simulink model "ROSCO_v1"  (R2023a)
settings: Solver=ode4  StartTime=0.0  StopTime=TMax  FixedStep=simu.dt  RelTol=1e-3  EnableMultiTasking=on
undefined symbols (not defined in the file): Azimuth_list, DiscIntNeverNeededParam, F, n_FixFrameInputs, n_FixFrameOutputs, n_RotTripletInputs, n_RotTripletOutputs, new_seq_inp, new_seq_out, OutList, Parameter, R, rpm2radps, simu, StateSpace, strmatch
libraries: simulink x10
(part 2 of 3)

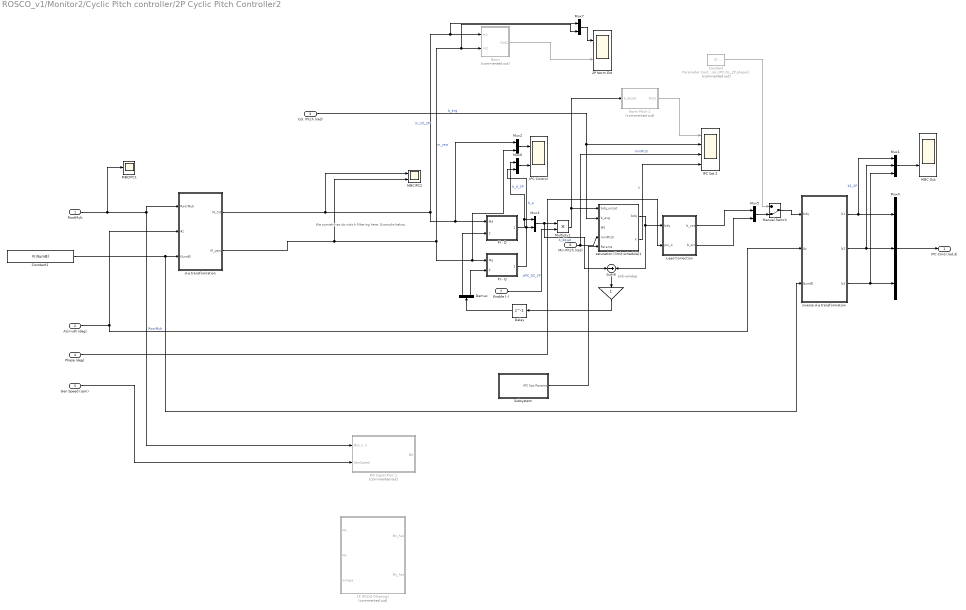
== system ROSCO_v1/Monitor2/Cyclic Pitch controller/2P Cyclic Pitch Controller2 ==
  note: We sometimes do notch filtering here. Example below.
  note: anti-windup
  note: k
  RootMyb : Inport
  Azimuth (deg) : Inport  Port=2
  Col. Pitch (rad) : Inport  Port=3
  Phase (deg) : Inport  Port=4
  Gen Speed (rpm) : Inport  Port=5
  Min Pitch (rad) : Inport  Port=6
  Enable (-) : Inport  Port=7
  " " : Gain
  1P IPCDQ Filtering1 : Subsystem  Commented=on
  2P Norm Est : Scope  NumInputPorts=2
  Constant : Constant  Commented=on  Value=Parameter.Control.cIPC.OL_2P.amp * [cosd(Parameter.Control.cIPC.OL_2P.phase), sind(Parameter.Control.cIPC.OL_2P.phase)]
  Constant1 : Constant  Value=R.NumBl
  Delay : Delay  DelayLength=1
  Demux : Demux  Outputs=2
  IPC Control : Scope  NumInputPorts=2
  IPC Sat 2 : Scope  NumInputPorts=4
  Lead Correction : MATLAB Function  TreatAsAtomicUnit=on
  M0 Signal Proc.1 : Subsystem  Commented=on
  MBC Out : Scope  NumInputPorts=2
  MBCIPC1 : Scope
  MBCIPC2 : Scope  NumInputPorts=2
  Manual Switch : ManualSwitch  CurrentSetting=0
  Multiply1 : Product
  Mux1 : Mux  Inputs=3
  Mux{2..3,5..7} (5 alike) : Mux  Inputs=2
  Mux4 : Mux  Inputs=3
  Norm : Subsystem  Commented=on
  Norm Pitch 2 : Subsystem  Commented=on
  PI - D : Subsystem  TreatAsAtomicUnit=on  SystemSampleTime=simu.dt
      settings: MinAlgLoopOccurrences=on
  PI - Q : Subsystem  TreatAsAtomicUnit=on  SystemSampleTime=simu.dt
      settings: MinAlgLoopOccurrences=on
  Subsystem : Subsystem
  Sum9 : Sum  Inputs=-|+
  d-q transformation : MATLAB Function  TreatAsAtomicUnit=on
  inverse d-q transformation : MATLAB Function  TreatAsAtomicUnit=on
  saturation (limit schedule)1 : MATLAB Function  TreatAsAtomicUnit=on
  IPC Cmd (rad,3) : Outport  VectorParamsAs1DForOutWhenUnconnected=off
  wires:
  Enable (-)/1 -> Multiply1/2  "cIPC_GS_2P"
  Norm Pitch 2/1(Out1) -> IPC Sat 2/1
  Min Pitch (rad)/1 -> saturation (limit schedule)1/4(minPitch), IPC Sat 2/3  "minPitch"
  Norm/1(Out1) -> 2P Norm Est/2
  Mux7/1 -> 2P Norm Est/1
  Mux2/1 -> IPC Control/1
  Mux6/1 -> IPC Control/2
  Mux1/1 -> MBC Out/2
  d-q transformation/2(M_yaw) -> PI - Q/1(Mq), Mux2/2, Norm/2(In2), Mux7/2, MBCIPC2/2  "m_yaw"
  Constant1/1 -> inverse d-q transformation/3(NumBl), d-q transformation/3(NumBl)
  saturation (limit schedule)1/2(k) -> IPC Sat 2/4
  Lead Correction/2(b_sin) -> Mux5/2
  Lead Correction/1(b_cos) -> Mux5/1
  Azimuth (deg)/1 -> inverse d-q transformation/2(Az), d-q transformation/2(Az)
  Sum9/1 -> " "/1
  RootMyb/1 -> MBCIPC1/1, M0 Signal Proc.1/1("My1,2, 3"), d-q transformation/1(RootMyb)  "RootMyb"
  " "/1 -> Delay/1
  Delay/1 -> Demux/1
  Mux4/1 -> IPC Cmd (rad,3)/1
  inverse d-q transformation/2(b2) -> Mux4/2, Mux1/2
  Demux/2 -> PI - Q/2(Anti-windup)
  inverse d-q transformation/1(b1) -> Mux4/1, Mux1/1  "b1_2P"
  Demux/1 -> PI - D/2(Anti-windup)
  PI - D/1(Theta_tilt) -> Mux6/1, Mux3/1  "b_d_2P"
  PI - Q/1(Theta_yaw) -> Mux6/2, Mux3/2  "b_q"
  Phase (deg)/1 -> Lead Correction/2(psi_o)
  inverse d-q transformation/3(b3) -> Mux4/3, Mux1/3
  d-q transformation/1(M_tilt) -> PI - D/1(Md), Mux2/1, Norm/1(In1), Mux7/1, MBCIPC2/1  "m_tilt_2P"
  Gen Speed (rpm)/1 -> M0 Signal Proc.1/2(GenSpeed)
  saturation (limit schedule)1/1(bdq) -> Lead Correction/1(bdq), Sum9/2
  Col. Pitch (rad)/1 -> IPC Sat 2/2, saturation (limit schedule)1/2(b_avg)  "b_avg"
  Subsystem/1(IPC Sat Params) -> saturation (limit schedule)1/5(Params)
  Mux3/1 -> Sum9/1, Multiply1/1  "b_dqsat"
  Multiply1/1 -> Norm Pitch 2/1(b_dqsat), saturation (limit schedule)1/1(bdq_unsat)
  Mux5/1 -> Manual Switch/2
  Manual Switch/1 -> inverse d-q transformation/1(bdq)
  Constant/1 -> Manual Switch/1

== system ROSCO_v1/Torque Controller/VS_OmegaRef/Omega_opt ==
  note: % Assuming known wind speed, initially, and not using GenSpeed
  TSR_opt : Inport
  Wind Speed : Inport  Port=2
  Divide : Product  Inputs=*/
  Multiply : Product
  "Rot -> GenSpeed" : Gain  Gain=R.GBRatio
  Rotor Radius : Constant  Value=R.RotorRad
  Omega_opt : Outport  VectorParamsAs1DForOutWhenUnconnected=off
  wires:
  TSR_opt/1 -> Multiply/1
  Wind Speed/1 -> Multiply/2
  Multiply/1 -> Divide/1
  Rotor Radius/1 -> Divide/2
  Divide/1 -> "Rot -> GenSpeed"/1
  "Rot -> GenSpeed"/1 -> Omega_opt/1

== system ROSCO_v1/Monitor2/Cyclic Pitch controller/1P Cyclic Pitch Controller1/1P IPCDQ Filtering1 ==
  Mx : Inport
  My : Inport  Port=2
  omega : Inport  Port=3
  Discrete Filter2 : DiscreteFilter  Numerator=Parameter.Control.cIPC.IPCDQ_LPF.Numerator{1}  Denominator=Parameter.Control.cIPC.IPCDQ_LPF.Denominator{1}  SampleTime=Parameter.Control.DT
  Discrete Filter3 : DiscreteFilter  Numerator=Parameter.Control.cIPC.IPCDQ_LPF.Numerator{1}  Denominator=Parameter.Control.cIPC.IPCDQ_LPF.Denominator{1}  SampleTime=Parameter.Control.DT
  IPC NFs Man 2 : Scope  NumInputPorts=2
  Moving 3P Notch Man Y : Subsystem
  Moving 3P Notch Man Z : Subsystem
  Moving 6P Notch Man Y : Subsystem
  Moving 6P Notch Man Z : Subsystem
  Mux : Mux  Inputs=2
  Mux1 : Mux  Inputs=2
  Mx_hat : Outport  VectorParamsAs1DForOutWhenUnconnected=off
  My_hat : Outport  Port=2  VectorParamsAs1DForOutWhenUnconnected=off
  wires:
  omega/1 -> Moving 6P Notch Man Y/2(GenSpeedIN), Moving 3P Notch Man Y/2(GenSpeedIN), Moving 6P Notch Man Z/2(GenSpeedIN), Moving 3P Notch Man Z/2(GenSpeedIN)
  Mx/1 -> Mux/1, Moving 3P Notch Man Y/1(Input)
  My/1 -> Mux1/1, Moving 3P Notch Man Z/1(Input)
  Moving 6P Notch Man Z/1(Output) -> Discrete Filter3/1
  Moving 6P Notch Man Y/1(Output) -> Discrete Filter2/1
  Moving 3P Notch Man Y/1(Output) -> Moving 6P Notch Man Y/1(Input)
  Moving 3P Notch Man Z/1(Output) -> Moving 6P Notch Man Z/1(Input)
  Mux1/1 -> IPC NFs Man 2/2
  Mux/1 -> IPC NFs Man 2/1
  Discrete Filter3/1 -> Mux1/2, My_hat/1
  Discrete Filter2/1 -> Mux/2, Mx_hat/1

== system ROSCO_v1/Monitor2/Cyclic Pitch controller/1P Cyclic Pitch Controller1/M0 Signal Proc.1 ==
  "My1,2, 3" : Inport
  GenSpeed : Inport  Port=2
  Add : Sum  Inputs=+++
  Demux1 : Demux  Outputs=3
  Discrete Filter : DiscreteFilter  Numerator=Parameter.Control.cIPC.PSM0_LPF.Numerator{1}  Denominator=Parameter.Control.cIPC.PSM0_LPF.Denominator{1}  a0EqualsOne=on
  Gain : Gain  Gain=1/3
  Moving 1P Notch Man : Subsystem
  Moving 3P Notch Man : Subsystem
  Mux : Mux  Inputs=2
  Scope : Scope  NumInputPorts=2
  M0 : Outport  VectorParamsAs1DForOutWhenUnconnected=off
  wires:
  Demux1/1 -> Add/1
  Demux1/2 -> Add/2
  Add/1 -> Gain/1
  "My1,2, 3"/1 -> Demux1/1
  GenSpeed/1 -> Moving 3P Notch Man/2(GenSpeedIN), Moving 1P Notch Man/2(GenSpeedIN)
  Demux1/3 -> Add/3
  Moving 1P Notch Man/1(Output) -> Moving 3P Notch Man/1(Input)
  Mux/1 -> Scope/2
  Gain/1 -> Scope/1, Moving 1P Notch Man/1(Input)
  Moving 3P Notch Man/1(Output) -> Discrete Filter/1
  Discrete Filter/1 -> Mux/1, M0/1

== system ROSCO_v1/Monitor2/Cyclic Pitch controller/1P Cyclic Pitch Controller1/Norm ==
  In1 : Inport
  In2 : Inport  Port=2
  Add : Sum
  Discrete Filter1 : DiscreteFilter  Numerator=Parameter.Control.cIPC.IPCDQ_LPF.num{1}  Denominator=Parameter.Control.cIPC.IPCDQ_LPF.den{1}  SampleTime=Parameter.Control.DT
  Product : Product
  Product1 : Product
  Sqrt : Sqrt
  Out1 : Outport  VectorParamsAs1DForOutWhenUnconnected=off
  wires:
  Product/1 -> Add/1
  Product1/1 -> Add/2
  Sqrt/1 -> Discrete Filter1/1
  Add/1 -> Sqrt/1
  In2/1 -> Product1/1, Product1/2
  In1/1 -> Product/1, Product/2
  Discrete Filter1/1 -> Out1/1

== system ROSCO_v1/Monitor2/Cyclic Pitch controller/1P Cyclic Pitch Controller1/Norm Pitch ==
  b_dqsat : Inport
  Demux1 : Demux  Outputs=2
  Sqrt : Sqrt
  Square : Math  Operator=square  SignedPower=on
  Square1 : Math  Operator=square  SignedPower=on
  Sum : Sum
  Out1 : Outport  VectorParamsAs1DForOutWhenUnconnected=off
  wires:
  Demux1/1 -> Square/1
  Square1/1 -> Sum/2
  b_dqsat/1 -> Demux1/1
  Sum/1 -> Sqrt/1
  Demux1/2 -> Square1/1
  Square/1 -> Sum/1
  Sqrt/1 -> Out1/1

== system ROSCO_v1/Monitor2/Cyclic Pitch controller/1P Cyclic Pitch Controller1/PI - D ==
  Md : Inport
  Anti-windup : Inport  Port=2
  Discrete Derivative : simulink/Discrete/Discrete Derivative  gainval=1.0  ICPrevScaledInput=0.0  OutMin=[]  OutMax=[]  OutDataType=fixdt(1, 16)  OutScaling=2^-10  DoSatur=off
  Discrete Filter1 : DiscreteFilter  Commented=through  Numerator=Parameter.Control.cIPC.IPCDQ_LPF.num{1}  Denominator=Parameter.Control.cIPC.IPCDQ_LPF.den{1}  SampleTime=Parameter.Control.DT
  Integrator : DiscreteIntegrator  IntegratorMethod=Integration: Backward Euler  gainval=1  SampleTime=simu.dt  UpperSaturationLimit=1.570796/(.008068634/9.5492966)/(1./(1.+pi/2/.109997))  LowerSaturationLimit=0  ICPrevOutput=DiscIntNeverNeededParam  ICPrevScaledInput=DiscIntNeverNeededParam
  Kd : Gain  Gain=0
  Ki : Gain  Gain=R.IPC_KI_2P
  Kp : Gain  Gain=R.IPC_KP_1P
  Scope : Scope  NumInputPorts=2
  Sum3 : Sum  Inputs=+++
  Sum8 : Sum  Inputs=|++
  Theta_tilt : Outport  VectorParamsAs1DForOutWhenUnconnected=off
  wires:
  Ki/1 -> Sum8/1
  Sum3/1 -> Scope/1, Theta_tilt/1
  Md/1 -> Ki/1, Kp/1, Discrete Filter1/1
  Anti-windup/1 -> Scope/2, Sum8/2
  Sum8/1 -> Integrator/1
  Kd/1 -> Discrete Derivative/1
  Kp/1 -> Sum3/2
  Discrete Derivative/1 -> Sum3/1
  Integrator/1 -> Sum3/3
  Discrete Filter1/1 -> Kd/1

== system ROSCO_v1/Monitor2/Cyclic Pitch controller/1P Cyclic Pitch Controller1/PI - Q ==
  Mq : Inport
  Anti-windup : Inport  Port=2
  Discrete Derivative : simulink/Discrete/Discrete Derivative  gainval=1.0  ICPrevScaledInput=0.0  OutMin=[]  OutMax=[]  OutDataType=fixdt(1, 16)  OutScaling=2^-10  DoSatur=off
  Discrete Filter1 : DiscreteFilter  Commented=through  Numerator=Parameter.Control.cIPC.IPCDQ_LPF.num{1}  Denominator=Parameter.Control.cIPC.IPCDQ_LPF.den{1}  SampleTime=Parameter.Control.DT
  Integrator1 : DiscreteIntegrator  IntegratorMethod=Integration: Backward Euler  gainval=1  SampleTime=simu.dt  UpperSaturationLimit=1.570796/(.008068634/9.5492966)/(1./(1.+pi/2/.109997))  LowerSaturationLimit=0  ICPrevOutput=DiscIntNeverNeededParam  ICPrevScaledInput=DiscIntNeverNeededParam
  Kd : Gain  Gain=0
  Ki : Gain  Gain=R.IPC_KI_1P
  Kp : Gain  Gain=R.IPC_KP_1P
  Sum10 : Sum  Inputs=|++
  Sum3 : Sum  Inputs=+++
  Theta_yaw : Outport  VectorParamsAs1DForOutWhenUnconnected=off
  wires:
  Sum3/1 -> Theta_yaw/1
  Sum10/1 -> Integrator1/1
  Anti-windup/1 -> Sum10/2
  Integrator1/1 -> Sum3/3
  Ki/1 -> Sum10/1
  Kp/1 -> Sum3/2
  Mq/1 -> Discrete Filter1/1, Kp/1, Ki/1
  Kd/1 -> Discrete Derivative/1
  Discrete Derivative/1 -> Sum3/1
  Discrete Filter1/1 -> Kd/1

== system ROSCO_v1/Monitor2/Cyclic Pitch controller/1P Cyclic Pitch Controller1/Subsystem1 ==
  Constant3 : Constant
  Constant4 : Constant  Value=0
  Constant5 : Constant  Value=0
  Mux : Mux  Inputs=3
  IPC Sat Params : Outport  VectorParamsAs1DForOutWhenUnconnected=off
  wires:
  Constant3/1 -> Mux/1
  Constant4/1 -> Mux/2
  Constant5/1 -> Mux/3
  Mux/1 -> IPC Sat Params/1

== system ROSCO_v1/Monitor2/Cyclic Pitch controller/2P Cyclic Pitch Controller2/1P IPCDQ Filtering1 ==
  Mx : Inport
  My : Inport  Port=2
  omega : Inport  Port=3
  Discrete Filter2 : DiscreteFilter  Numerator=Parameter.Control.cIPC.IPCDQ_LPF.Numerator{1}  Denominator=Parameter.Control.cIPC.IPCDQ_LPF.Denominator{1}  SampleTime=Parameter.Control.DT
  Discrete Filter3 : DiscreteFilter  Numerator=Parameter.Control.cIPC.IPCDQ_LPF.Numerator{1}  Denominator=Parameter.Control.cIPC.IPCDQ_LPF.Denominator{1}  SampleTime=Parameter.Control.DT
  IPC NFs Man 2 : Scope  NumInputPorts=2
  Moving 3P Notch Man Y : Subsystem
  Moving 3P Notch Man Z : Subsystem
  Moving 6P Notch Man Y : Subsystem
  Moving 6P Notch Man Z : Subsystem
  Mux : Mux  Inputs=2
  Mux1 : Mux  Inputs=2
  Mx_hat : Outport  VectorParamsAs1DForOutWhenUnconnected=off
  My_hat : Outport  Port=2  VectorParamsAs1DForOutWhenUnconnected=off
  wires:
  omega/1 -> Moving 6P Notch Man Y/2(GenSpeedIN), Moving 3P Notch Man Y/2(GenSpeedIN), Moving 6P Notch Man Z/2(GenSpeedIN), Moving 3P Notch Man Z/2(GenSpeedIN)
  Mx/1 -> Mux/1, Moving 3P Notch Man Y/1(Input)
  My/1 -> Mux1/1, Moving 3P Notch Man Z/1(Input)
  Moving 6P Notch Man Z/1(Output) -> Discrete Filter3/1
  Moving 6P Notch Man Y/1(Output) -> Discrete Filter2/1
  Moving 3P Notch Man Y/1(Output) -> Moving 6P Notch Man Y/1(Input)
  Moving 3P Notch Man Z/1(Output) -> Moving 6P Notch Man Z/1(Input)
  Mux1/1 -> IPC NFs Man 2/2
  Mux/1 -> IPC NFs Man 2/1
  Discrete Filter3/1 -> Mux1/2, My_hat/1
  Discrete Filter2/1 -> Mux/2, Mx_hat/1

== system ROSCO_v1/Monitor2/Cyclic Pitch controller/2P Cyclic Pitch Controller2/M0 Signal Proc.1 ==
  "My1,2, 3" : Inport
  GenSpeed : Inport  Port=2
  Add : Sum  Inputs=+++
  Demux1 : Demux  Outputs=3
  Discrete Filter : DiscreteFilter  Numerator=Parameter.Control.cIPC.PSM0_LPF.Numerator{1}  Denominator=Parameter.Control.cIPC.PSM0_LPF.Denominator{1}  a0EqualsOne=on
  Gain : Gain  Gain=1/3
  Moving 1P Notch Man : Subsystem
  Moving 3P Notch Man : Subsystem
  Mux : Mux  Inputs=2
  Scope : Scope  NumInputPorts=2
  M0 : Outport  VectorParamsAs1DForOutWhenUnconnected=off
  wires:
  Demux1/1 -> Add/1
  Demux1/2 -> Add/2
  Add/1 -> Gain/1
  "My1,2, 3"/1 -> Demux1/1
  GenSpeed/1 -> Moving 3P Notch Man/2(GenSpeedIN), Moving 1P Notch Man/2(GenSpeedIN)
  Demux1/3 -> Add/3
  Moving 1P Notch Man/1(Output) -> Moving 3P Notch Man/1(Input)
  Mux/1 -> Scope/2
  Gain/1 -> Scope/1, Moving 1P Notch Man/1(Input)
  Moving 3P Notch Man/1(Output) -> Discrete Filter/1
  Discrete Filter/1 -> Mux/1, M0/1

== system ROSCO_v1/Monitor2/Cyclic Pitch controller/2P Cyclic Pitch Controller2/Norm ==
  In1 : Inport
  In2 : Inport  Port=2
  Add : Sum
  Discrete Filter1 : DiscreteFilter  Numerator=Parameter.Control.cIPC.IPCDQ_LPF.num{1}  Denominator=Parameter.Control.cIPC.IPCDQ_LPF.den{1}  SampleTime=Parameter.Control.DT
  Product : Product
  Product1 : Product
  Sqrt : Sqrt
  Out1 : Outport  VectorParamsAs1DForOutWhenUnconnected=off
  wires:
  Discrete Filter1/1 -> Out1/1
  In1/1 -> Product/2, Product/1
  In2/1 -> Product1/2, Product1/1
  Add/1 -> Sqrt/1
  Sqrt/1 -> Discrete Filter1/1
  Product1/1 -> Add/2
  Product/1 -> Add/1

== system ROSCO_v1/Monitor2/Cyclic Pitch controller/2P Cyclic Pitch Controller2/Norm Pitch 2 ==
  b_dqsat : Inport
  Demux1 : Demux  Outputs=2
  Sqrt : Sqrt
  Square : Math  Operator=square  SignedPower=on
  Square1 : Math  Operator=square  SignedPower=on
  Sum : Sum
  Out1 : Outport  VectorParamsAs1DForOutWhenUnconnected=off
  wires:
  Sqrt/1 -> Out1/1
  Square/1 -> Sum/1
  Demux1/2 -> Square1/1
  Sum/1 -> Sqrt/1
  b_dqsat/1 -> Demux1/1
  Square1/1 -> Sum/2
  Demux1/1 -> Square/1

== system ROSCO_v1/Monitor2/Cyclic Pitch controller/2P Cyclic Pitch Controller2/PI - D ==
  Md : Inport
  Anti-windup : Inport  Port=2
  Discrete Derivative : simulink/Discrete/Discrete Derivative  gainval=1.0  ICPrevScaledInput=0.0  OutMin=[]  OutMax=[]  OutDataType=fixdt(1, 16)  OutScaling=2^-10  DoSatur=off
  Discrete Filter1 : DiscreteFilter  Commented=through  Numerator=Parameter.Control.cIPC.IPCDQ_LPF.num{1}  Denominator=Parameter.Control.cIPC.IPCDQ_LPF.den{1}  SampleTime=Parameter.Control.DT
  Integrator : DiscreteIntegrator  IntegratorMethod=Integration: Backward Euler  gainval=1  SampleTime=simu.dt  UpperSaturationLimit=1.570796/(.008068634/9.5492966)/(1./(1.+pi/2/.109997))  LowerSaturationLimit=0  ICPrevOutput=DiscIntNeverNeededParam  ICPrevScaledInput=DiscIntNeverNeededParam
  Kd : Gain  Gain=0
  Ki : Gain  Gain=R.IPC_KI_2P
  Kp : Gain  Gain=R.IPC_KP_2P
  Sum3 : Sum  Inputs=+++
  Sum8 : Sum  Inputs=|++
  Theta_tilt : Outport  VectorParamsAs1DForOutWhenUnconnected=off
  wires:
  Discrete Filter1/1 -> Kd/1
  Integrator/1 -> Sum3/3
  Discrete Derivative/1 -> Sum3/1
  Kp/1 -> Sum3/2
  Kd/1 -> Discrete Derivative/1
  Sum8/1 -> Integrator/1
  Anti-windup/1 -> Sum8/2
  Md/1 -> Discrete Filter1/1, Kp/1, Ki/1
  Sum3/1 -> Theta_tilt/1
  Ki/1 -> Sum8/1

== system ROSCO_v1/Monitor2/Cyclic Pitch controller/2P Cyclic Pitch Controller2/PI - Q ==
  Mq : Inport
  Anti-windup : Inport  Port=2
  Discrete Derivative : simulink/Discrete/Discrete Derivative  gainval=1.0  ICPrevScaledInput=0.0  OutMin=[]  OutMax=[]  OutDataType=fixdt(1, 16)  OutScaling=2^-10  DoSatur=off
  Discrete Filter1 : DiscreteFilter  Commented=through  Numerator=Parameter.Control.cIPC.IPCDQ_LPF.num{1}  Denominator=Parameter.Control.cIPC.IPCDQ_LPF.den{1}  SampleTime=Parameter.Control.DT
  Integrator1 : DiscreteIntegrator  IntegratorMethod=Integration: Backward Euler  gainval=1  SampleTime=simu.dt  UpperSaturationLimit=1.570796/(.008068634/9.5492966)/(1./(1.+pi/2/.109997))  LowerSaturationLimit=0  ICPrevOutput=DiscIntNeverNeededParam  ICPrevScaledInput=DiscIntNeverNeededParam
  Kd : Gain  Gain=0
  Ki : Gain  Gain=R.IPC_KI_2P
  Kp : Gain  Gain=R.IPC_KP_2P
  Sum10 : Sum  Inputs=|++
  Sum3 : Sum  Inputs=+++
  Theta_yaw : Outport  VectorParamsAs1DForOutWhenUnconnected=off
  wires:
  Discrete Filter1/1 -> Kd/1
  Discrete Derivative/1 -> Sum3/1
  Kd/1 -> Discrete Derivative/1
  Mq/1 -> Ki/1, Kp/1, Discrete Filter1/1
  Kp/1 -> Sum3/2
  Ki/1 -> Sum10/1
  Integrator1/1 -> Sum3/3
  Anti-windup/1 -> Sum10/2
  Sum10/1 -> Integrator1/1
  Sum3/1 -> Theta_yaw/1

== system ROSCO_v1/Monitor2/Cyclic Pitch controller/2P Cyclic Pitch Controller2/Subsystem ==
  Constant3 : Constant
  Constant4 : Constant  Value=0
  Constant5 : Constant  Value=0
  Mux : Mux  Inputs=3
  IPC Sat Params : Outport  VectorParamsAs1DForOutWhenUnconnected=off
  wires:
  Constant3/1 -> Mux/1
  Constant4/1 -> Mux/2
  Constant5/1 -> Mux/3
  Mux/1 -> IPC Sat Params/1

== system ROSCO_v1/Monitor2/Cyclic Pitch controller/1P Cyclic Pitch Controller1/1P IPCDQ Filtering1/Moving 3P Notch Man Y ==
  Input : Inport
  GenSpeedIN : Inport  Port=2
  Gain : Gain  Gain=1/Parameter.Turbine.G * rpm2radps(1) * 3
  Moving 3P Filt Manual : Subsystem
  Slow Low Pass for Param : DiscreteStateSpace  A=Parameter.Control.cIPC.dLPF_slow.a  B=Parameter.Control.cIPC.dLPF_slow.b  C=Parameter.Control.cIPC.dLPF_slow.c  D=Parameter.Control.cIPC.dLPF_slow.d  SampleTime=Parameter.Control.DT
  Output : Outport  VectorParamsAs1DForOutWhenUnconnected=off
  wires:
  Slow Low Pass for Param/1 -> Gain/1
  Gain/1 -> Moving 3P Filt Manual/2(rot speed (rad/s))
  Input/1 -> Moving 3P Filt Manual/1(u)
  GenSpeedIN/1 -> Slow Low Pass for Param/1
  Moving 3P Filt Manual/1(Out1) -> Output/1

== system ROSCO_v1/Monitor2/Cyclic Pitch controller/1P Cyclic Pitch Controller1/1P IPCDQ Filtering1/Moving 3P Notch Man Z ==
  Input : Inport
  GenSpeedIN : Inport  Port=2
  Gain : Gain  Gain=1/Parameter.Turbine.G * rpm2radps(1) * 3
  Moving 3P Filt Manual : Subsystem
  Slow Low Pass for Param : DiscreteStateSpace  A=Parameter.Control.cIPC.dLPF_slow.a  B=Parameter.Control.cIPC.dLPF_slow.b  C=Parameter.Control.cIPC.dLPF_slow.c  D=Parameter.Control.cIPC.dLPF_slow.d  SampleTime=Parameter.Control.DT
  Output : Outport  VectorParamsAs1DForOutWhenUnconnected=off
  wires:
  Moving 3P Filt Manual/1(Out1) -> Output/1
  GenSpeedIN/1 -> Slow Low Pass for Param/1
  Input/1 -> Moving 3P Filt Manual/1(u)
  Gain/1 -> Moving 3P Filt Manual/2(rot speed (rad/s))
  Slow Low Pass for Param/1 -> Gain/1

== system ROSCO_v1/Monitor2/Cyclic Pitch controller/1P Cyclic Pitch Controller1/1P IPCDQ Filtering1/Moving 6P Notch Man Y ==
  Input : Inport
  GenSpeedIN : Inport  Port=2
  Gain : Gain  Gain=1/Parameter.Turbine.G * rpm2radps(1) * 3
  Moving 6P Filt Manual : Subsystem
  Slow Low Pass for Param : DiscreteStateSpace  A=Parameter.Control.cIPC.dLPF_slow.a  B=Parameter.Control.cIPC.dLPF_slow.b  C=Parameter.Control.cIPC.dLPF_slow.c  D=Parameter.Control.cIPC.dLPF_slow.d  SampleTime=Parameter.Control.DT
  Output : Outport  VectorParamsAs1DForOutWhenUnconnected=off
  wires:
  Moving 6P Filt Manual/1(Out1) -> Output/1
  GenSpeedIN/1 -> Slow Low Pass for Param/1
  Input/1 -> Moving 6P Filt Manual/1(u)
  Gain/1 -> Moving 6P Filt Manual/2(rot speed (rad/s))
  Slow Low Pass for Param/1 -> Gain/1

== system ROSCO_v1/Monitor2/Cyclic Pitch controller/1P Cyclic Pitch Controller1/1P IPCDQ Filtering1/Moving 6P Notch Man Z ==
  Input : Inport
  GenSpeedIN : Inport  Port=2
  Gain : Gain  Gain=1/Parameter.Turbine.G * rpm2radps(1) * 3
  Moving 6P Filt Manual : Subsystem
  Slow Low Pass for Param : DiscreteStateSpace  A=Parameter.Control.cIPC.dLPF_slow.a  B=Parameter.Control.cIPC.dLPF_slow.b  C=Parameter.Control.cIPC.dLPF_slow.c  D=Parameter.Control.cIPC.dLPF_slow.d  SampleTime=Parameter.Control.DT
  Output : Outport  VectorParamsAs1DForOutWhenUnconnected=off
  wires:
  Slow Low Pass for Param/1 -> Gain/1
  Gain/1 -> Moving 6P Filt Manual/2(rot speed (rad/s))
  Input/1 -> Moving 6P Filt Manual/1(u)
  GenSpeedIN/1 -> Slow Low Pass for Param/1
  Moving 6P Filt Manual/1(Out1) -> Output/1

== system ROSCO_v1/Monitor2/Cyclic Pitch controller/1P Cyclic Pitch Controller1/M0 Signal Proc.1/Moving 1P Notch Man ==
  Input : Inport
  GenSpeedIN : Inport  Port=2
  Gain : Gain  Gain=1/Parameter.Turbine.G * rpm2radps(1)
  Moving 1P Filt Manual : Subsystem
  Slow Low Pass for Param : DiscreteStateSpace  A=Parameter.Control.cIPC.dLPF_slow.a  B=Parameter.Control.cIPC.dLPF_slow.b  C=Parameter.Control.cIPC.dLPF_slow.c  D=Parameter.Control.cIPC.dLPF_slow.d  SampleTime=Parameter.Control.DT
  Output : Outport  VectorParamsAs1DForOutWhenUnconnected=off
  wires:
  GenSpeedIN/1 -> Slow Low Pass for Param/1
  Input/1 -> Moving 1P Filt Manual/1(u)
  Gain/1 -> Moving 1P Filt Manual/2(rot speed (rad/s))
  Slow Low Pass for Param/1 -> Gain/1
  Moving 1P Filt Manual/1(Out1) -> Output/1

== system ROSCO_v1/Monitor2/Cyclic Pitch controller/1P Cyclic Pitch Controller1/M0 Signal Proc.1/Moving 3P Notch Man ==
  Input : Inport
  GenSpeedIN : Inport  Port=2
  Gain : Gain  Gain=1/Parameter.Turbine.G * rpm2radps(1) * 3
  Moving 3P Filt Manual : Subsystem
  Slow Low Pass for Param : DiscreteStateSpace  A=Parameter.Control.cIPC.dLPF_slow.a  B=Parameter.Control.cIPC.dLPF_slow.b  C=Parameter.Control.cIPC.dLPF_slow.c  D=Parameter.Control.cIPC.dLPF_slow.d  SampleTime=Parameter.Control.DT
  Output : Outport  VectorParamsAs1DForOutWhenUnconnected=off
  wires:
  Slow Low Pass for Param/1 -> Gain/1
  Gain/1 -> Moving 3P Filt Manual/2(rot speed (rad/s))
  Input/1 -> Moving 3P Filt Manual/1(u)
  GenSpeedIN/1 -> Slow Low Pass for Param/1
  Moving 3P Filt Manual/1(Out1) -> Output/1

== system ROSCO_v1/Monitor2/Cyclic Pitch controller/2P Cyclic Pitch Controller2/1P IPCDQ Filtering1/Moving 3P Notch Man Y ==
  Input : Inport
  GenSpeedIN : Inport  Port=2
  Gain : Gain  Gain=1/Parameter.Turbine.G * rpm2radps(1) * 3
  Moving 3P Filt Manual : Subsystem
  Slow Low Pass for Param : DiscreteStateSpace  A=Parameter.Control.cIPC.dLPF_slow.a  B=Parameter.Control.cIPC.dLPF_slow.b  C=Parameter.Control.cIPC.dLPF_slow.c  D=Parameter.Control.cIPC.dLPF_slow.d  SampleTime=Parameter.Control.DT
  Output : Outport  VectorParamsAs1DForOutWhenUnconnected=off
  wires:
  Slow Low Pass for Param/1 -> Gain/1
  Gain/1 -> Moving 3P Filt Manual/2(rot speed (rad/s))
  Input/1 -> Moving 3P Filt Manual/1(u)
  GenSpeedIN/1 -> Slow Low Pass for Param/1
  Moving 3P Filt Manual/1(Out1) -> Output/1

== system ROSCO_v1/Monitor2/Cyclic Pitch controller/2P Cyclic Pitch Controller2/1P IPCDQ Filtering1/Moving 3P Notch Man Z ==
  Input : Inport
  GenSpeedIN : Inport  Port=2
  Gain : Gain  Gain=1/Parameter.Turbine.G * rpm2radps(1) * 3
  Moving 3P Filt Manual : Subsystem
  Slow Low Pass for Param : DiscreteStateSpace  A=Parameter.Control.cIPC.dLPF_slow.a  B=Parameter.Control.cIPC.dLPF_slow.b  C=Parameter.Control.cIPC.dLPF_slow.c  D=Parameter.Control.cIPC.dLPF_slow.d  SampleTime=Parameter.Control.DT
  Output : Outport  VectorParamsAs1DForOutWhenUnconnected=off
  wires:
  Moving 3P Filt Manual/1(Out1) -> Output/1
  GenSpeedIN/1 -> Slow Low Pass for Param/1
  Input/1 -> Moving 3P Filt Manual/1(u)
  Gain/1 -> Moving 3P Filt Manual/2(rot speed (rad/s))
  Slow Low Pass for Param/1 -> Gain/1

== system ROSCO_v1/Monitor2/Cyclic Pitch controller/2P Cyclic Pitch Controller2/1P IPCDQ Filtering1/Moving 6P Notch Man Y ==
  Input : Inport
  GenSpeedIN : Inport  Port=2
  Gain : Gain  Gain=1/Parameter.Turbine.G * rpm2radps(1) * 3
  Moving 6P Filt Manual : Subsystem
  Slow Low Pass for Param : DiscreteStateSpace  A=Parameter.Control.cIPC.dLPF_slow.a  B=Parameter.Control.cIPC.dLPF_slow.b  C=Parameter.Control.cIPC.dLPF_slow.c  D=Parameter.Control.cIPC.dLPF_slow.d  SampleTime=Parameter.Control.DT
  Output : Outport  VectorParamsAs1DForOutWhenUnconnected=off
  wires:
  Moving 6P Filt Manual/1(Out1) -> Output/1
  GenSpeedIN/1 -> Slow Low Pass for Param/1
  Input/1 -> Moving 6P Filt Manual/1(u)
  Gain/1 -> Moving 6P Filt Manual/2(rot speed (rad/s))
  Slow Low Pass for Param/1 -> Gain/1

== system ROSCO_v1/Monitor2/Cyclic Pitch controller/2P Cyclic Pitch Controller2/1P IPCDQ Filtering1/Moving 6P Notch Man Z ==
  Input : Inport
  GenSpeedIN : Inport  Port=2
  Gain : Gain  Gain=1/Parameter.Turbine.G * rpm2radps(1) * 3
  Moving 6P Filt Manual : Subsystem
  Slow Low Pass for Param : DiscreteStateSpace  A=Parameter.Control.cIPC.dLPF_slow.a  B=Parameter.Control.cIPC.dLPF_slow.b  C=Parameter.Control.cIPC.dLPF_slow.c  D=Parameter.Control.cIPC.dLPF_slow.d  SampleTime=Parameter.Control.DT
  Output : Outport  VectorParamsAs1DForOutWhenUnconnected=off
  wires:
  Slow Low Pass for Param/1 -> Gain/1
  Gain/1 -> Moving 6P Filt Manual/2(rot speed (rad/s))
  Input/1 -> Moving 6P Filt Manual/1(u)
  GenSpeedIN/1 -> Slow Low Pass for Param/1
  Moving 6P Filt Manual/1(Out1) -> Output/1

== system ROSCO_v1/Monitor2/Cyclic Pitch controller/2P Cyclic Pitch Controller2/M0 Signal Proc.1/Moving 1P Notch Man ==
  Input : Inport
  GenSpeedIN : Inport  Port=2
  Gain : Gain  Gain=1/Parameter.Turbine.G * rpm2radps(1)
  Moving 1P Filt Manual : Subsystem
  Slow Low Pass for Param : DiscreteStateSpace  A=Parameter.Control.cIPC.dLPF_slow.a  B=Parameter.Control.cIPC.dLPF_slow.b  C=Parameter.Control.cIPC.dLPF_slow.c  D=Parameter.Control.cIPC.dLPF_slow.d  SampleTime=Parameter.Control.DT
  Output : Outport  VectorParamsAs1DForOutWhenUnconnected=off
  wires:
  GenSpeedIN/1 -> Slow Low Pass for Param/1
  Input/1 -> Moving 1P Filt Manual/1(u)
  Gain/1 -> Moving 1P Filt Manual/2(rot speed (rad/s))
  Slow Low Pass for Param/1 -> Gain/1
  Moving 1P Filt Manual/1(Out1) -> Output/1

== system ROSCO_v1/Monitor2/Cyclic Pitch controller/2P Cyclic Pitch Controller2/M0 Signal Proc.1/Moving 3P Notch Man ==
  Input : Inport
  GenSpeedIN : Inport  Port=2
  Gain : Gain  Gain=1/Parameter.Turbine.G * rpm2radps(1) * 3
  Moving 3P Filt Manual : Subsystem
  Slow Low Pass for Param : DiscreteStateSpace  A=Parameter.Control.cIPC.dLPF_slow.a  B=Parameter.Control.cIPC.dLPF_slow.b  C=Parameter.Control.cIPC.dLPF_slow.c  D=Parameter.Control.cIPC.dLPF_slow.d  SampleTime=Parameter.Control.DT
  Output : Outport  VectorParamsAs1DForOutWhenUnconnected=off
  wires:
  Slow Low Pass for Param/1 -> Gain/1
  Gain/1 -> Moving 3P Filt Manual/2(rot speed (rad/s))
  Input/1 -> Moving 3P Filt Manual/1(u)
  GenSpeedIN/1 -> Slow Low Pass for Param/1
  Moving 3P Filt Manual/1(Out1) -> Output/1

== system ROSCO_v1/Monitor2/Cyclic Pitch controller/1P Cyclic Pitch Controller1/1P IPCDQ Filtering1/Moving 3P Notch Man Y/Moving 3P Filt Manual ==
  u : Inport
  rot speed (rad/s) : Inport  Port=2
  Den LPV : Subsystem
  Discrete Filter : DiscreteFilter  NumeratorSource=Input port  DenominatorSource=Input port  a0EqualsOne=on
      settings: InputPortMap=u0,p1,p3
  Num LPV : Subsystem
  Out1 : Outport  VectorParamsAs1DForOutWhenUnconnected=off
  wires:
  u/1 -> Discrete Filter/1
  Num LPV/1(b) -> Discrete Filter/2
  Discrete Filter/1 -> Out1/1
  rot speed (rad/s)/1 -> Den LPV/1(rot speed (rad/s)), Num LPV/1(rot speed (rad/s))
  Den LPV/1(a) -> Discrete Filter/3

== system ROSCO_v1/Monitor2/Cyclic Pitch controller/1P Cyclic Pitch Controller1/1P IPCDQ Filtering1/Moving 3P Notch Man Z/Moving 3P Filt Manual ==
  u : Inport
  rot speed (rad/s) : Inport  Port=2
  Den LPV : Subsystem
  Discrete Filter : DiscreteFilter  NumeratorSource=Input port  DenominatorSource=Input port  a0EqualsOne=on
      settings: InputPortMap=u0,p1,p3
  Num LPV : Subsystem
  Out1 : Outport  VectorParamsAs1DForOutWhenUnconnected=off
  wires:
  Den LPV/1(a) -> Discrete Filter/3
  rot speed (rad/s)/1 -> Num LPV/1(rot speed (rad/s)), Den LPV/1(rot speed (rad/s))
  Discrete Filter/1 -> Out1/1
  Num LPV/1(b) -> Discrete Filter/2
  u/1 -> Discrete Filter/1

== system ROSCO_v1/Monitor2/Cyclic Pitch controller/1P Cyclic Pitch Controller1/1P IPCDQ Filtering1/Moving 6P Notch Man Y/Moving 6P Filt Manual ==
  u : Inport
  rot speed (rad/s) : Inport  Port=2
  Den LPV : Subsystem
  Discrete Filter : DiscreteFilter  NumeratorSource=Input port  DenominatorSource=Input port  a0EqualsOne=on
      settings: InputPortMap=u0,p1,p3
  Num LPV : Subsystem
  Out1 : Outport  VectorParamsAs1DForOutWhenUnconnected=off
  wires:
  Den LPV/1(a) -> Discrete Filter/3
  rot speed (rad/s)/1 -> Num LPV/1(rot speed (rad/s)), Den LPV/1(rot speed (rad/s))
  Discrete Filter/1 -> Out1/1
  Num LPV/1(b) -> Discrete Filter/2
  u/1 -> Discrete Filter/1

== system ROSCO_v1/Monitor2/Cyclic Pitch controller/1P Cyclic Pitch Controller1/1P IPCDQ Filtering1/Moving 6P Notch Man Z/Moving 6P Filt Manual ==
  u : Inport
  rot speed (rad/s) : Inport  Port=2
  Den LPV : Subsystem
  Discrete Filter : DiscreteFilter  NumeratorSource=Input port  DenominatorSource=Input port  a0EqualsOne=on
      settings: InputPortMap=u0,p1,p3
  Num LPV : Subsystem
  Out1 : Outport  VectorParamsAs1DForOutWhenUnconnected=off
  wires:
  u/1 -> Discrete Filter/1
  Num LPV/1(b) -> Discrete Filter/2
  Discrete Filter/1 -> Out1/1
  rot speed (rad/s)/1 -> Den LPV/1(rot speed (rad/s)), Num LPV/1(rot speed (rad/s))
  Den LPV/1(a) -> Discrete Filter/3

== system ROSCO_v1/Monitor2/Cyclic Pitch controller/1P Cyclic Pitch Controller1/M0 Signal Proc.1/Moving 1P Notch Man/Moving 1P Filt Manual ==
  u : Inport
  rot speed (rad/s) : Inport  Port=2
  Den LPV : Subsystem
  Discrete Filter : DiscreteFilter  NumeratorSource=Input port  DenominatorSource=Input port  a0EqualsOne=on
      settings: InputPortMap=u0,p1,p3
  Num LPV : Subsystem
  Out1 : Outport  VectorParamsAs1DForOutWhenUnconnected=off
  wires:
  Den LPV/1(a) -> Discrete Filter/3
  rot speed (rad/s)/1 -> Num LPV/1(rot speed (rad/s)), Den LPV/1(rot speed (rad/s))
  Discrete Filter/1 -> Out1/1
  Num LPV/1(b) -> Discrete Filter/2
  u/1 -> Discrete Filter/1

== system ROSCO_v1/Monitor2/Cyclic Pitch controller/1P Cyclic Pitch Controller1/M0 Signal Proc.1/Moving 3P Notch Man/Moving 3P Filt Manual ==
  u : Inport
  rot speed (rad/s) : Inport  Port=2
  Den LPV : Subsystem
  Discrete Filter : DiscreteFilter  NumeratorSource=Input port  DenominatorSource=Input port  a0EqualsOne=on
      settings: InputPortMap=u0,p1,p3
  Num LPV : Subsystem
  Out1 : Outport  VectorParamsAs1DForOutWhenUnconnected=off
  wires:
  u/1 -> Discrete Filter/1
  Num LPV/1(b) -> Discrete Filter/2
  Discrete Filter/1 -> Out1/1
  rot speed (rad/s)/1 -> Den LPV/1(rot speed (rad/s)), Num LPV/1(rot speed (rad/s))
  Den LPV/1(a) -> Discrete Filter/3

== system ROSCO_v1/Monitor2/Cyclic Pitch controller/2P Cyclic Pitch Controller2/1P IPCDQ Filtering1/Moving 3P Notch Man Y/Moving 3P Filt Manual ==
  u : Inport
  rot speed (rad/s) : Inport  Port=2
  Den LPV : Subsystem
  Discrete Filter : DiscreteFilter  NumeratorSource=Input port  DenominatorSource=Input port  a0EqualsOne=on
      settings: InputPortMap=u0,p1,p3
  Num LPV : Subsystem
  Out1 : Outport  VectorParamsAs1DForOutWhenUnconnected=off
  wires:
  u/1 -> Discrete Filter/1
  Num LPV/1(b) -> Discrete Filter/2
  Discrete Filter/1 -> Out1/1
  rot speed (rad/s)/1 -> Den LPV/1(rot speed (rad/s)), Num LPV/1(rot speed (rad/s))
  Den LPV/1(a) -> Discrete Filter/3

== system ROSCO_v1/Monitor2/Cyclic Pitch controller/2P Cyclic Pitch Controller2/1P IPCDQ Filtering1/Moving 3P Notch Man Z/Moving 3P Filt Manual ==
  u : Inport
  rot speed (rad/s) : Inport  Port=2
  Den LPV : Subsystem
  Discrete Filter : DiscreteFilter  NumeratorSource=Input port  DenominatorSource=Input port  a0EqualsOne=on
      settings: InputPortMap=u0,p1,p3
  Num LPV : Subsystem
  Out1 : Outport  VectorParamsAs1DForOutWhenUnconnected=off
  wires:
  Den LPV/1(a) -> Discrete Filter/3
  rot speed (rad/s)/1 -> Num LPV/1(rot speed (rad/s)), Den LPV/1(rot speed (rad/s))
  Discrete Filter/1 -> Out1/1
  Num LPV/1(b) -> Discrete Filter/2
  u/1 -> Discrete Filter/1

== system ROSCO_v1/Monitor2/Cyclic Pitch controller/2P Cyclic Pitch Controller2/1P IPCDQ Filtering1/Moving 6P Notch Man Y/Moving 6P Filt Manual ==
  u : Inport
  rot speed (rad/s) : Inport  Port=2
  Den LPV : Subsystem
  Discrete Filter : DiscreteFilter  NumeratorSource=Input port  DenominatorSource=Input port  a0EqualsOne=on
      settings: InputPortMap=u0,p1,p3
  Num LPV : Subsystem
  Out1 : Outport  VectorParamsAs1DForOutWhenUnconnected=off
  wires:
  Den LPV/1(a) -> Discrete Filter/3
  rot speed (rad/s)/1 -> Num LPV/1(rot speed (rad/s)), Den LPV/1(rot speed (rad/s))
  Discrete Filter/1 -> Out1/1
  Num LPV/1(b) -> Discrete Filter/2
  u/1 -> Discrete Filter/1

== system ROSCO_v1/Monitor2/Cyclic Pitch controller/2P Cyclic Pitch Controller2/1P IPCDQ Filtering1/Moving 6P Notch Man Z/Moving 6P Filt Manual ==
  u : Inport
  rot speed (rad/s) : Inport  Port=2
  Den LPV : Subsystem
  Discrete Filter : DiscreteFilter  NumeratorSource=Input port  DenominatorSource=Input port  a0EqualsOne=on
      settings: InputPortMap=u0,p1,p3
  Num LPV : Subsystem
  Out1 : Outport  VectorParamsAs1DForOutWhenUnconnected=off
  wires:
  u/1 -> Discrete Filter/1
  Num LPV/1(b) -> Discrete Filter/2
  Discrete Filter/1 -> Out1/1
  rot speed (rad/s)/1 -> Den LPV/1(rot speed (rad/s)), Num LPV/1(rot speed (rad/s))
  Den LPV/1(a) -> Discrete Filter/3

== system ROSCO_v1/Monitor2/Cyclic Pitch controller/2P Cyclic Pitch Controller2/M0 Signal Proc.1/Moving 1P Notch Man/Moving 1P Filt Manual ==
  u : Inport
  rot speed (rad/s) : Inport  Port=2
  Den LPV : Subsystem
  Discrete Filter : DiscreteFilter  NumeratorSource=Input port  DenominatorSource=Input port  a0EqualsOne=on
      settings: InputPortMap=u0,p1,p3
  Num LPV : Subsystem
  Out1 : Outport  VectorParamsAs1DForOutWhenUnconnected=off
  wires:
  Den LPV/1(a) -> Discrete Filter/3
  rot speed (rad/s)/1 -> Num LPV/1(rot speed (rad/s)), Den LPV/1(rot speed (rad/s))
  Discrete Filter/1 -> Out1/1
  Num LPV/1(b) -> Discrete Filter/2
  u/1 -> Discrete Filter/1

== system ROSCO_v1/Monitor2/Cyclic Pitch controller/2P Cyclic Pitch Controller2/M0 Signal Proc.1/Moving 3P Notch Man/Moving 3P Filt Manual ==
  u : Inport
  rot speed (rad/s) : Inport  Port=2
  Den LPV : Subsystem
  Discrete Filter : DiscreteFilter  NumeratorSource=Input port  DenominatorSource=Input port  a0EqualsOne=on
      settings: InputPortMap=u0,p1,p3
  Num LPV : Subsystem
  Out1 : Outport  VectorParamsAs1DForOutWhenUnconnected=off
  wires:
  u/1 -> Discrete Filter/1
  Num LPV/1(b) -> Discrete Filter/2
  Discrete Filter/1 -> Out1/1
  rot speed (rad/s)/1 -> Den LPV/1(rot speed (rad/s)), Num LPV/1(rot speed (rad/s))
  Den LPV/1(a) -> Discrete Filter/3

== system ROSCO_v1/Monitor2/Cyclic Pitch controller/1P Cyclic Pitch Controller1/1P IPCDQ Filtering1/Moving 3P Notch Man Y/Moving 3P Filt Manual/Den LPV ==
  rot speed (rad/s) : Inport
  1-D Lookup Table : Lookup_n-D  NumberOfTableDimensions=1  BreakpointsForDimension1=Parameter.Control.cIPC.PSM0_NF_3P.om_3P  BeginIndexSearchUsingPreviousIndexResult=on  Table=Parameter.Control.cIPC.PSM0_NF_3P.a_2  ExtrapMethod=Clip  InternalRulePriority=Speed  RndMeth=Simplest
  1-D Lookup Table1 : Lookup_n-D  NumberOfTableDimensions=1  BreakpointsForDimension1=Parameter.Control.cIPC.PSM0_NF_3P.om_3P  BeginIndexSearchUsingPreviousIndexResult=on  Table=Parameter.Control.cIPC.PSM0_NF_3P.a_1  ExtrapMethod=Clip  InternalRulePriority=Speed  RndMeth=Simplest
  1-D Lookup Table2 : Lookup_n-D  NumberOfTableDimensions=1  BreakpointsForDimension1=Parameter.Control.cIPC.PSM0_NF_3P.om_3P  BeginIndexSearchUsingPreviousIndexResult=on  Table=Parameter.Control.cIPC.PSM0_NF_3P.a_0  ExtrapMethod=Clip  InternalRulePriority=Speed  RndMeth=Simplest
  Mux : Mux  Inputs=3
  a : Outport  VectorParamsAs1DForOutWhenUnconnected=off
  wires:
  1-D Lookup Table/1 -> Mux/1
  1-D Lookup Table1/1 -> Mux/2
  Mux/1 -> a/1
  rot speed (rad/s)/1 -> 1-D Lookup Table2/1, 1-D Lookup Table/1, 1-D Lookup Table1/1
  1-D Lookup Table2/1 -> Mux/3

== system ROSCO_v1/Monitor2/Cyclic Pitch controller/1P Cyclic Pitch Controller1/1P IPCDQ Filtering1/Moving 3P Notch Man Y/Moving 3P Filt Manual/Num LPV ==
  rot speed (rad/s) : Inport
  1-D Lookup Table : Lookup_n-D  NumberOfTableDimensions=1  BreakpointsForDimension1=Parameter.Control.cIPC.PSM0_NF_3P.om_3P  BeginIndexSearchUsingPreviousIndexResult=on  Table=Parameter.Control.cIPC.PSM0_NF_3P.b_2  ExtrapMethod=Clip  InternalRulePriority=Speed  RndMeth=Simplest
  1-D Lookup Table1 : Lookup_n-D  NumberOfTableDimensions=1  BreakpointsForDimension1=Parameter.Control.cIPC.PSM0_NF_3P.om_3P  BeginIndexSearchUsingPreviousIndexResult=on  Table=Parameter.Control.cIPC.PSM0_NF_3P.b_1  ExtrapMethod=Clip  InternalRulePriority=Speed  RndMeth=Simplest
  1-D Lookup Table2 : Lookup_n-D  NumberOfTableDimensions=1  BreakpointsForDimension1=Parameter.Control.cIPC.PSM0_NF_3P.om_3P  BeginIndexSearchUsingPreviousIndexResult=on  Table=Parameter.Control.cIPC.PSM0_NF_3P.b_0  ExtrapMethod=Clip  InternalRulePriority=Speed  RndMeth=Simplest
  Mux : Mux  Inputs=3
  b : Outport  VectorParamsAs1DForOutWhenUnconnected=off
  wires:
  1-D Lookup Table2/1 -> Mux/3
  rot speed (rad/s)/1 -> 1-D Lookup Table1/1, 1-D Lookup Table/1, 1-D Lookup Table2/1
  Mux/1 -> b/1
  1-D Lookup Table1/1 -> Mux/2
  1-D Lookup Table/1 -> Mux/1

== system ROSCO_v1/Monitor2/Cyclic Pitch controller/1P Cyclic Pitch Controller1/1P IPCDQ Filtering1/Moving 3P Notch Man Z/Moving 3P Filt Manual/Den LPV ==
  rot speed (rad/s) : Inport
  1-D Lookup Table : Lookup_n-D  NumberOfTableDimensions=1  BreakpointsForDimension1=Parameter.Control.cIPC.PSM0_NF_3P.om_3P  BeginIndexSearchUsingPreviousIndexResult=on  Table=Parameter.Control.cIPC.PSM0_NF_3P.a_2  ExtrapMethod=Clip  InternalRulePriority=Speed  RndMeth=Simplest
  1-D Lookup Table1 : Lookup_n-D  NumberOfTableDimensions=1  BreakpointsForDimension1=Parameter.Control.cIPC.PSM0_NF_3P.om_3P  BeginIndexSearchUsingPreviousIndexResult=on  Table=Parameter.Control.cIPC.PSM0_NF_3P.a_1  ExtrapMethod=Clip  InternalRulePriority=Speed  RndMeth=Simplest
  1-D Lookup Table2 : Lookup_n-D  NumberOfTableDimensions=1  BreakpointsForDimension1=Parameter.Control.cIPC.PSM0_NF_3P.om_3P  BeginIndexSearchUsingPreviousIndexResult=on  Table=Parameter.Control.cIPC.PSM0_NF_3P.a_0  ExtrapMethod=Clip  InternalRulePriority=Speed  RndMeth=Simplest
  Mux : Mux  Inputs=3
  a : Outport  VectorParamsAs1DForOutWhenUnconnected=off
  wires:
  1-D Lookup Table2/1 -> Mux/3
  rot speed (rad/s)/1 -> 1-D Lookup Table1/1, 1-D Lookup Table/1, 1-D Lookup Table2/1
  Mux/1 -> a/1
  1-D Lookup Table1/1 -> Mux/2
  1-D Lookup Table/1 -> Mux/1

== system ROSCO_v1/Monitor2/Cyclic Pitch controller/1P Cyclic Pitch Controller1/1P IPCDQ Filtering1/Moving 3P Notch Man Z/Moving 3P Filt Manual/Num LPV ==
  rot speed (rad/s) : Inport
  1-D Lookup Table : Lookup_n-D  NumberOfTableDimensions=1  BreakpointsForDimension1=Parameter.Control.cIPC.PSM0_NF_3P.om_3P  BeginIndexSearchUsingPreviousIndexResult=on  Table=Parameter.Control.cIPC.PSM0_NF_3P.b_2  ExtrapMethod=Clip  InternalRulePriority=Speed  RndMeth=Simplest
  1-D Lookup Table1 : Lookup_n-D  NumberOfTableDimensions=1  BreakpointsForDimension1=Parameter.Control.cIPC.PSM0_NF_3P.om_3P  BeginIndexSearchUsingPreviousIndexResult=on  Table=Parameter.Control.cIPC.PSM0_NF_3P.b_1  ExtrapMethod=Clip  InternalRulePriority=Speed  RndMeth=Simplest
  1-D Lookup Table2 : Lookup_n-D  NumberOfTableDimensions=1  BreakpointsForDimension1=Parameter.Control.cIPC.PSM0_NF_3P.om_3P  BeginIndexSearchUsingPreviousIndexResult=on  Table=Parameter.Control.cIPC.PSM0_NF_3P.b_0  ExtrapMethod=Clip  InternalRulePriority=Speed  RndMeth=Simplest
  Mux : Mux  Inputs=3
  b : Outport  VectorParamsAs1DForOutWhenUnconnected=off
  wires:
  1-D Lookup Table/1 -> Mux/1
  1-D Lookup Table1/1 -> Mux/2
  Mux/1 -> b/1
  rot speed (rad/s)/1 -> 1-D Lookup Table2/1, 1-D Lookup Table/1, 1-D Lookup Table1/1
  1-D Lookup Table2/1 -> Mux/3

== system ROSCO_v1/Monitor2/Cyclic Pitch controller/1P Cyclic Pitch Controller1/1P IPCDQ Filtering1/Moving 6P Notch Man Y/Moving 6P Filt Manual/Den LPV ==
  rot speed (rad/s) : Inport
  1-D Lookup Table : Lookup_n-D  NumberOfTableDimensions=1  BreakpointsForDimension1=Parameter.Control.cIPC.PSM0_NF_6P.om_6P  BeginIndexSearchUsingPreviousIndexResult=on  Table=Parameter.Control.cIPC.PSM0_NF_6P.a_2  ExtrapMethod=Clip  InternalRulePriority=Speed  RndMeth=Simplest
  1-D Lookup Table1 : Lookup_n-D  NumberOfTableDimensions=1  BreakpointsForDimension1=Parameter.Control.cIPC.PSM0_NF_6P.om_6P  BeginIndexSearchUsingPreviousIndexResult=on  Table=Parameter.Control.cIPC.PSM0_NF_6P.a_1  ExtrapMethod=Clip  InternalRulePriority=Speed  RndMeth=Simplest
  1-D Lookup Table2 : Lookup_n-D  NumberOfTableDimensions=1  BreakpointsForDimension1=Parameter.Control.cIPC.PSM0_NF_6P.om_6P  BeginIndexSearchUsingPreviousIndexResult=on  Table=Parameter.Control.cIPC.PSM0_NF_6P.a_0  ExtrapMethod=Clip  InternalRulePriority=Speed  RndMeth=Simplest
  Mux : Mux  Inputs=3
  a : Outport  VectorParamsAs1DForOutWhenUnconnected=off
  wires:
  1-D Lookup Table2/1 -> Mux/3
  rot speed (rad/s)/1 -> 1-D Lookup Table1/1, 1-D Lookup Table/1, 1-D Lookup Table2/1
  Mux/1 -> a/1
  1-D Lookup Table1/1 -> Mux/2
  1-D Lookup Table/1 -> Mux/1

== system ROSCO_v1/Monitor2/Cyclic Pitch controller/1P Cyclic Pitch Controller1/1P IPCDQ Filtering1/Moving 6P Notch Man Y/Moving 6P Filt Manual/Num LPV ==
  rot speed (rad/s) : Inport
  1-D Lookup Table : Lookup_n-D  NumberOfTableDimensions=1  BreakpointsForDimension1=Parameter.Control.cIPC.PSM0_NF_6P.om_6P  BeginIndexSearchUsingPreviousIndexResult=on  Table=Parameter.Control.cIPC.PSM0_NF_6P.b_2  ExtrapMethod=Clip  InternalRulePriority=Speed  RndMeth=Simplest
  1-D Lookup Table1 : Lookup_n-D  NumberOfTableDimensions=1  BreakpointsForDimension1=Parameter.Control.cIPC.PSM0_NF_6P.om_6P  BeginIndexSearchUsingPreviousIndexResult=on  Table=Parameter.Control.cIPC.PSM0_NF_6P.b_1  ExtrapMethod=Clip  InternalRulePriority=Speed  RndMeth=Simplest
  1-D Lookup Table2 : Lookup_n-D  NumberOfTableDimensions=1  BreakpointsForDimension1=Parameter.Control.cIPC.PSM0_NF_6P.om_6P  BeginIndexSearchUsingPreviousIndexResult=on  Table=Parameter.Control.cIPC.PSM0_NF_6P.b_0  ExtrapMethod=Clip  InternalRulePriority=Speed  RndMeth=Simplest
  Mux : Mux  Inputs=3
  b : Outport  VectorParamsAs1DForOutWhenUnconnected=off
  wires:
  1-D Lookup Table/1 -> Mux/1
  1-D Lookup Table1/1 -> Mux/2
  Mux/1 -> b/1
  rot speed (rad/s)/1 -> 1-D Lookup Table2/1, 1-D Lookup Table1/1, 1-D Lookup Table/1
  1-D Lookup Table2/1 -> Mux/3

== system ROSCO_v1/Monitor2/Cyclic Pitch controller/1P Cyclic Pitch Controller1/1P IPCDQ Filtering1/Moving 6P Notch Man Z/Moving 6P Filt Manual/Den LPV ==
  rot speed (rad/s) : Inport
  1-D Lookup Table : Lookup_n-D  NumberOfTableDimensions=1  BreakpointsForDimension1=Parameter.Control.cIPC.PSM0_NF_6P.om_6P  BeginIndexSearchUsingPreviousIndexResult=on  Table=Parameter.Control.cIPC.PSM0_NF_6P.a_2  ExtrapMethod=Clip  InternalRulePriority=Speed  RndMeth=Simplest
  1-D Lookup Table1 : Lookup_n-D  NumberOfTableDimensions=1  BreakpointsForDimension1=Parameter.Control.cIPC.PSM0_NF_6P.om_6P  BeginIndexSearchUsingPreviousIndexResult=on  Table=Parameter.Control.cIPC.PSM0_NF_6P.a_1  ExtrapMethod=Clip  InternalRulePriority=Speed  RndMeth=Simplest
  1-D Lookup Table2 : Lookup_n-D  NumberOfTableDimensions=1  BreakpointsForDimension1=Parameter.Control.cIPC.PSM0_NF_6P.om_6P  BeginIndexSearchUsingPreviousIndexResult=on  Table=Parameter.Control.cIPC.PSM0_NF_6P.a_0  ExtrapMethod=Clip  InternalRulePriority=Speed  RndMeth=Simplest
  Mux : Mux  Inputs=3
  a : Outport  VectorParamsAs1DForOutWhenUnconnected=off
  wires:
  1-D Lookup Table/1 -> Mux/1
  1-D Lookup Table1/1 -> Mux/2
  Mux/1 -> a/1
  rot speed (rad/s)/1 -> 1-D Lookup Table2/1, 1-D Lookup Table/1, 1-D Lookup Table1/1
  1-D Lookup Table2/1 -> Mux/3

== system ROSCO_v1/Monitor2/Cyclic Pitch controller/1P Cyclic Pitch Controller1/1P IPCDQ Filtering1/Moving 6P Notch Man Z/Moving 6P Filt Manual/Num LPV ==
  rot speed (rad/s) : Inport
  1-D Lookup Table : Lookup_n-D  NumberOfTableDimensions=1  BreakpointsForDimension1=Parameter.Control.cIPC.PSM0_NF_6P.om_6P  BeginIndexSearchUsingPreviousIndexResult=on  Table=Parameter.Control.cIPC.PSM0_NF_6P.b_2  ExtrapMethod=Clip  InternalRulePriority=Speed  RndMeth=Simplest
  1-D Lookup Table1 : Lookup_n-D  NumberOfTableDimensions=1  BreakpointsForDimension1=Parameter.Control.cIPC.PSM0_NF_6P.om_6P  BeginIndexSearchUsingPreviousIndexResult=on  Table=Parameter.Control.cIPC.PSM0_NF_6P.b_1  ExtrapMethod=Clip  InternalRulePriority=Speed  RndMeth=Simplest
  1-D Lookup Table2 : Lookup_n-D  NumberOfTableDimensions=1  BreakpointsForDimension1=Parameter.Control.cIPC.PSM0_NF_6P.om_6P  BeginIndexSearchUsingPreviousIndexResult=on  Table=Parameter.Control.cIPC.PSM0_NF_6P.b_0  ExtrapMethod=Clip  InternalRulePriority=Speed  RndMeth=Simplest
  Mux : Mux  Inputs=3
  b : Outport  VectorParamsAs1DForOutWhenUnconnected=off
  wires:
  1-D Lookup Table2/1 -> Mux/3
  rot speed (rad/s)/1 -> 1-D Lookup Table1/1, 1-D Lookup Table/1, 1-D Lookup Table2/1
  Mux/1 -> b/1
  1-D Lookup Table1/1 -> Mux/2
  1-D Lookup Table/1 -> Mux/1

== system ROSCO_v1/Monitor2/Cyclic Pitch controller/1P Cyclic Pitch Controller1/M0 Signal Proc.1/Moving 1P Notch Man/Moving 1P Filt Manual/Den LPV ==
  rot speed (rad/s) : Inport
  1-D Lookup Table : Lookup_n-D  NumberOfTableDimensions=1  BreakpointsForDimension1=Parameter.Control.cIPC.PSM0_NF_1P.om_1P  BeginIndexSearchUsingPreviousIndexResult=on  Table=Parameter.Control.cIPC.PSM0_NF_1P.a_2  ExtrapMethod=Clip  InternalRulePriority=Speed  RndMeth=Simplest
  1-D Lookup Table1 : Lookup_n-D  NumberOfTableDimensions=1  BreakpointsForDimension1=Parameter.Control.cIPC.PSM0_NF_1P.om_1P  BeginIndexSearchUsingPreviousIndexResult=on  Table=Parameter.Control.cIPC.PSM0_NF_1P.a_1  ExtrapMethod=Clip  InternalRulePriority=Speed  RndMeth=Simplest
  1-D Lookup Table2 : Lookup_n-D  NumberOfTableDimensions=1  BreakpointsForDimension1=Parameter.Control.cIPC.PSM0_NF_1P.om_1P  BeginIndexSearchUsingPreviousIndexResult=on  Table=Parameter.Control.cIPC.PSM0_NF_1P.a_0  ExtrapMethod=Clip  InternalRulePriority=Speed  RndMeth=Simplest
  Mux : Mux  Inputs=3
  a : Outport  VectorParamsAs1DForOutWhenUnconnected=off
  wires:
  1-D Lookup Table2/1 -> Mux/3
  rot speed (rad/s)/1 -> 1-D Lookup Table1/1, 1-D Lookup Table/1, 1-D Lookup Table2/1
  Mux/1 -> a/1
  1-D Lookup Table1/1 -> Mux/2
  1-D Lookup Table/1 -> Mux/1

== system ROSCO_v1/Monitor2/Cyclic Pitch controller/1P Cyclic Pitch Controller1/M0 Signal Proc.1/Moving 1P Notch Man/Moving 1P Filt Manual/Num LPV ==
  rot speed (rad/s) : Inport
  1-D Lookup Table : Lookup_n-D  NumberOfTableDimensions=1  BreakpointsForDimension1=Parameter.Control.cIPC.PSM0_NF_1P.om_1P  BeginIndexSearchUsingPreviousIndexResult=on  Table=Parameter.Control.cIPC.PSM0_NF_1P.b_2  ExtrapMethod=Clip  InternalRulePriority=Speed  RndMeth=Simplest
  1-D Lookup Table1 : Lookup_n-D  NumberOfTableDimensions=1  BreakpointsForDimension1=Parameter.Control.cIPC.PSM0_NF_1P.om_1P  BeginIndexSearchUsingPreviousIndexResult=on  Table=Parameter.Control.cIPC.PSM0_NF_1P.b_1  ExtrapMethod=Clip  InternalRulePriority=Speed  RndMeth=Simplest
  1-D Lookup Table2 : Lookup_n-D  NumberOfTableDimensions=1  BreakpointsForDimension1=Parameter.Control.cIPC.PSM0_NF_1P.om_1P  BeginIndexSearchUsingPreviousIndexResult=on  Table=Parameter.Control.cIPC.PSM0_NF_1P.b_0  ExtrapMethod=Clip  InternalRulePriority=Speed  RndMeth=Simplest
  Mux : Mux  Inputs=3
  b : Outport  VectorParamsAs1DForOutWhenUnconnected=off
  wires:
  1-D Lookup Table/1 -> Mux/1
  1-D Lookup Table1/1 -> Mux/2
  Mux/1 -> b/1
  rot speed (rad/s)/1 -> 1-D Lookup Table2/1, 1-D Lookup Table/1, 1-D Lookup Table1/1
  1-D Lookup Table2/1 -> Mux/3

== system ROSCO_v1/Monitor2/Cyclic Pitch controller/1P Cyclic Pitch Controller1/M0 Signal Proc.1/Moving 3P Notch Man/Moving 3P Filt Manual/Den LPV ==
  rot speed (rad/s) : Inport
  1-D Lookup Table : Lookup_n-D  NumberOfTableDimensions=1  BreakpointsForDimension1=Parameter.Control.cIPC.PSM0_NF_3P.om_3P  BeginIndexSearchUsingPreviousIndexResult=on  Table=Parameter.Control.cIPC.PSM0_NF_3P.a_2  ExtrapMethod=Clip  InternalRulePriority=Speed  RndMeth=Simplest
  1-D Lookup Table1 : Lookup_n-D  NumberOfTableDimensions=1  BreakpointsForDimension1=Parameter.Control.cIPC.PSM0_NF_3P.om_3P  BeginIndexSearchUsingPreviousIndexResult=on  Table=Parameter.Control.cIPC.PSM0_NF_3P.a_1  ExtrapMethod=Clip  InternalRulePriority=Speed  RndMeth=Simplest
  1-D Lookup Table2 : Lookup_n-D  NumberOfTableDimensions=1  BreakpointsForDimension1=Parameter.Control.cIPC.PSM0_NF_3P.om_3P  BeginIndexSearchUsingPreviousIndexResult=on  Table=Parameter.Control.cIPC.PSM0_NF_3P.a_0  ExtrapMethod=Clip  InternalRulePriority=Speed  RndMeth=Simplest
  Mux : Mux  Inputs=3
  a : Outport  VectorParamsAs1DForOutWhenUnconnected=off
  wires:
  1-D Lookup Table/1 -> Mux/1
  1-D Lookup Table1/1 -> Mux/2
  Mux/1 -> a/1
  rot speed (rad/s)/1 -> 1-D Lookup Table2/1, 1-D Lookup Table/1, 1-D Lookup Table1/1
  1-D Lookup Table2/1 -> Mux/3
